simulink library "BESS_lib"  (Simulink 8.1)
settings: Solver=ode45  SolverMode=SingleTasking  StartTime=0.0  StopTime=10.0  RelTol=1e-3
undefined symbols (not defined in the file or in its folder): DiscIntNeverNeededParam, gcbh, sps_rtmsupport, Ts
libraries: simulink x25, powerlib x6, powerlib_meascontrol x4, powerlib_extras x3, simulink_extras x1, debounce_lib x1
(part 2 of 2)

== system BESS_lib/NREL_BESS/Protection/bitwise_faults ==
  note: Constant array has LSB on most left.
  S : Inport
  Bitwise Operator : simulink/Logic and Bit Operations/Bitwise Operator  logicop=OR  UseBitMask=off  NumInputPorts=8  BitMask=bin2dec('11011001')  BitMaskRealWorld=Stored Integer
  Data Type Conversion : DataTypeConversion  OutDataTypeStr=uint16
  Data Type Conversion1 : DataTypeConversion  OutDataTypeStr=double
  Demux : Demux  Outputs=8
  Shift Arithmetic : ArithShift  BitShiftNumber=1  BitShiftDirection=Left
  Shift Arithmetic1 : ArithShift  BitShiftNumber=2  BitShiftDirection=Left
  Shift Arithmetic2 : ArithShift  BitShiftNumber=3  BitShiftDirection=Left
  Shift Arithmetic3 : ArithShift  BitShiftNumber=4  BitShiftDirection=Left
  Shift Arithmetic4 : ArithShift  BitShiftNumber=5  BitShiftDirection=Left
  Shift Arithmetic5 : ArithShift  BitShiftNumber=6  BitShiftDirection=Left
  Shift Arithmetic6 : ArithShift  BitShiftNumber=7  BitShiftDirection=Left
  s : Outport
  wires:
  Shift Arithmetic6/1 -> Bitwise Operator/8
  Demux/8 -> Shift Arithmetic6/1
  Shift Arithmetic5/1 -> Bitwise Operator/7
  Shift Arithmetic4/1 -> Bitwise Operator/6
  Shift Arithmetic3/1 -> Bitwise Operator/5
  Shift Arithmetic2/1 -> Bitwise Operator/4
  Shift Arithmetic1/1 -> Bitwise Operator/3
  Shift Arithmetic/1 -> Bitwise Operator/2
  Demux/7 -> Shift Arithmetic5/1
  Demux/6 -> Shift Arithmetic4/1
  Demux/5 -> Shift Arithmetic3/1
  Demux/4 -> Shift Arithmetic2/1
  Demux/3 -> Shift Arithmetic1/1
  Demux/2 -> Shift Arithmetic/1
  Demux/1 -> Bitwise Operator/1
  Data Type Conversion1/1 -> s/1
  Bitwise Operator/1 -> Data Type Conversion1/1
  S/1 -> Data Type Conversion/1
  Data Type Conversion/1 -> Demux/1

== system BESS_lib/NREL_BESS/Protection/bitwise_status ==
  note: Constant array has LSB on most left.
  S : Inport
  Bitwise Operator : simulink/Logic and Bit Operations/Bitwise Operator  logicop=OR  UseBitMask=off  NumInputPorts=3  BitMask=bin2dec('11011001')  BitMaskRealWorld=Stored Integer
  Data Type Conversion : DataTypeConversion  OutDataTypeStr=uint16
  Data Type Conversion1 : DataTypeConversion  OutDataTypeStr=double
  Demux : Demux  Outputs=3
  Shift Arithmetic : ArithShift  BitShiftNumber=1  BitShiftDirection=Left
  Shift Arithmetic1 : ArithShift  BitShiftNumber=2  BitShiftDirection=Left
  s : Outport
  wires:
  Data Type Conversion/1 -> Demux/1
  S/1 -> Data Type Conversion/1
  Bitwise Operator/1 -> Data Type Conversion1/1
  Data Type Conversion1/1 -> s/1
  Demux/1 -> Bitwise Operator/1
  Demux/2 -> Shift Arithmetic/1
  Demux/3 -> Shift Arithmetic1/1
  Shift Arithmetic/1 -> Bitwise Operator/2
  Shift Arithmetic1/1 -> Bitwise Operator/3

== system BESS_lib/NREL_BESS/Ref_Limiting/RefLimiting ==
  fvpq_in : Inport
  p_max : Inport  Port=2
  p_min : Inport  Port=3
  Complex to Magnitude-Angle : ComplexToMagnitudeAngle
  Complex to Real-Imag : ComplexToRealImag
  Demux : Demux
  Magnitude-Angle to Complex : MagnitudeAngleToComplex
  Mux2 : Mux
  Real-Imag to Complex : RealImagToComplex
  Saturation : Saturate  UpperLimit=1.1  LowerLimit=0.9
  Saturation Dynamic : simulink/Discontinuities/Saturation Dynamic  OutMin=[]  OutMax=[]  OutDataTypeStr=Inherit: Same as second input  OutDataType=fixdt(1, 16)  OutScaling=2^-10  DoSatur=off
  Saturation1 : Saturate  UpperLimit=1.1  LowerLimit=0.9
  Saturation2 : Saturate  UpperLimit=1  LowerLimit=0
  fvpq_out : Outport
  wires:
  p_min/1 -> Saturation Dynamic/3
  Saturation1/1 -> Mux2/2
  Magnitude-Angle to Complex/1 -> Complex to Real-Imag/1
  Mux2/1 -> fvpq_out/1  "fvpq"
  Demux/3 -> Saturation Dynamic/2
  Saturation Dynamic/1 -> Real-Imag to Complex/1
  Complex to Magnitude-Angle/1 -> Saturation2/1
  Complex to Real-Imag/2 -> Mux2/4
  Complex to Real-Imag/1 -> Mux2/3
  Real-Imag to Complex/1 -> Complex to Magnitude-Angle/1
  Demux/2 -> Saturation1/1
  Demux/1 -> Saturation/1
  fvpq_in/1 -> Demux/1
  Saturation2/1 -> Magnitude-Angle to Complex/1
  Saturation/1 -> Mux2/1
  p_max/1 -> Saturation Dynamic/1
  Complex to Magnitude-Angle/2 -> Magnitude-Angle to Complex/2
  Demux/4 -> Real-Imag to Complex/2

== system BESS_lib/NREL_BESS/Inverter Controller/rate_limit/RateLimitwRst ==
  Rst : Inport
  In : Inport  Port=2
  Constant : Constant  Value=0
  Saturation : Saturate  UpperLimit=Ts*BP.I_slewrate  LowerLimit=-Ts*BP.I_slewrate
  Sum : Sum  Inputs=-+|
  Sum1 : Sum  Inputs=|++
  Switch : Switch  Criteria=u2 > Threshold  Threshold=0.5
  Unit Delay : UnitDelay  SampleTime=Ts
  Out : Outport
  wires:
  Sum1/1 -> Switch/3
  Saturation/1 -> Sum1/1
  Rst/1 -> Switch/2
  Switch/1 -> Unit Delay/1
  Constant/1 -> Switch/1
  Unit Delay/1 -> Out/1, Sum/1, Sum1/2
  Sum/1 -> Saturation/1
  In/1 -> Sum/2

== system BESS_lib/NREL_BESS/Inverter Controller/rate_limit/RateLimitwRst1 ==
  Rst : Inport
  In : Inport  Port=2
  Constant : Constant  Value=0
  Saturation : Saturate  UpperLimit=Ts*BP.I_slewrate  LowerLimit=-Ts*BP.I_slewrate
  Sum : Sum  Inputs=-+|
  Sum1 : Sum  Inputs=|++
  Switch : Switch  Criteria=u2 > Threshold  Threshold=0.5
  Unit Delay : UnitDelay  SampleTime=Ts
  Out : Outport
  wires:
  In/1 -> Sum/2
  Sum/1 -> Saturation/1
  Unit Delay/1 -> Sum1/2, Sum/1, Out/1
  Constant/1 -> Switch/1
  Switch/1 -> Unit Delay/1
  Rst/1 -> Switch/2
  Saturation/1 -> Sum1/1
  Sum1/1 -> Switch/3

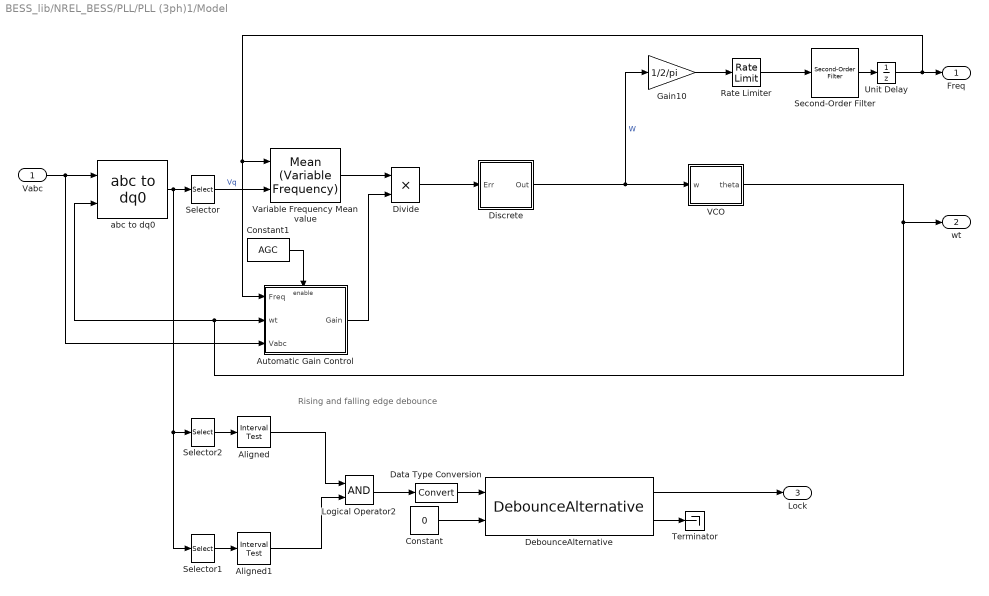
== system BESS_lib/NREL_BESS/PLL/PLL (3ph)1/Model ==
  note: Rising and falling edge debounce
  Vabc : Inport  PortDimensions=3
  Aligned : simulink/Logic and Bit Operations/Interval Test  IntervalClosedRight=on  uplimit=0.05  IntervalClosedLeft=on  lowlimit=-0.05  OutDataTypeStr=boolean
  Aligned1 : simulink/Logic and Bit Operations/Interval Test  IntervalClosedRight=on  uplimit=1.25  IntervalClosedLeft=on  lowlimit=0.05  OutDataTypeStr=boolean
  Automatic Gain Control : Subsystem  TreatAsAtomicUnit=on
  Constant : Constant  Value=0
  Constant1 : Constant  Value=AGC  SampleTime=Ts
  Data Type Conversion : DataTypeConversion
  DebounceAlternative : debounce_lib/DebounceAlternative  Tdb_off=0.5  Tdb_on=4  Tdb_sample=Tc
  Discrete : Subsystem  DialogController=POWERSYS.PowerSysDialog  VariantControl=PID_Discrete  mask(Discrete PID Controller){Kp=ParK(1), Ki=ParK(2), Kd=ParK(3), TcD=TcD, Par_Limits=[Flim(2) Flim(1)]*2*pi, Init=2*pi*Par_Init(2), Ts=Ts}
      mask prompts: Kp "Proportional gain (Kp):"; Ki "Integral gain (Ki):"; Kd "Derivative gain (Kd):"; TcD "Time constant for derivative filter (s):"; Par_Limits "Output limits: [ Upper   Lower ]"; Init "Output initial value:"; Ts "Sample time:"
      mask help: This block implements a discrete PID controller.
      mask Display: disp('PID');
  Divide : Product
  Gain10 : Gain  Gain=1/2/pi  SaturateOnIntegerOverflow=on  OutDataTypeStr=Inherit: Same as input  ParamDataTypeStr=Inherit: Same as input
  Logical Operator2 : Logic  AllPortsSameDT=off  OutDataTypeStr=boolean
  Rate Limiter : RateLimiter  RisingSlewLimit=MaxRateChangeFreq  FallingSlewLimit=-MaxRateChangeFreq  SampleTimeMode=inherited  InitialCondition=Par_Init(2)
  Second-Order Filter : powerlib_meascontrol/Filters/Second-Order Filter  FilterType=Lowpass  Fo=FilterCutOffFreq  Zeta=0.707  Ts=Ts  Initialize=on  Vac_Init=[0 0 Par_Init(2)]  Vdc_Init=Par_Init(2)  PlotResponse=off  FreqRange=[1 500 1]
  Selector : Selector  InputPortWidth=3  IndexOptions=Index vector (dialog)  Indices=2  OutputSizes=1
  Selector1 : Selector  InputPortWidth=3  IndexOptions=Index vector (dialog)  Indices=1  OutputSizes=1
  Selector2 : Selector  InputPortWidth=3  IndexOptions=Index vector (dialog)  Indices=2  OutputSizes=1
  Terminator : Terminator
  Unit Delay : UnitDelay  InitialCondition=Par_Init(2)  SampleTime=Ts
  VCO : Subsystem
  Variable Frequency Mean value : powerlib_meascontrol/Measurements/Mean (Variable Frequency)  Finit=Par_Init(2)  Fmin=Flim(1)  Vinit=0  Ts=Ts
  abc to dq0 : powerlib_meascontrol/Transformations/abc to dq0  Alignment=90 degrees behind phase A axis
  Freq : Outport
  wt : Outport  Port=2
  Lock : Outport  Port=3
  wires:
  VCO/1(theta) -> abc to dq0/2, Automatic Gain Control/2(wt), wt/1
  Data Type Conversion/1 -> DebounceAlternative/1
  Constant/1 -> DebounceAlternative/2
  DebounceAlternative/2 -> Terminator/1
  Logical Operator2/1 -> Data Type Conversion/1
  Selector2/1 -> Aligned/1
  Selector1/1 -> Aligned1/1
  Aligned1/1 -> Logical Operator2/2
  Aligned/1 -> Logical Operator2/1
  DebounceAlternative/1 -> Lock/1
  Discrete/1(Out) -> VCO/1(w), Gain10/1  "W"
  Unit Delay/1 -> Freq/1, Automatic Gain Control/1(Freq), Variable Frequency Mean value/1
  Rate Limiter/1 -> Second-Order Filter/1
  Gain10/1 -> Rate Limiter/1
  Selector/1 -> Variable Frequency Mean value/2  "Vq"
  Second-Order Filter/1 -> Unit Delay/1
  abc to dq0/1 -> Selector/1, Selector1/1, Selector2/1
  Vabc/1 -> abc to dq0/1, Automatic Gain Control/3(Vabc)
  Variable Frequency Mean value/1 -> Divide/1
  Automatic Gain Control/1(Gain) -> Divide/2
  Divide/1 -> Discrete/1(Err)
  Constant1/1 -> Automatic Gain Control/Enable

== system BESS_lib/NREL_BESS/Protection/Fault_Latch/SR_Prior_S ==
  S : Inport
  R : Inport  Port=2
  Logical Operator2 : Logic  Operator=OR  AllPortsSameDT=off  OutDataTypeStr=boolean
  Logical Operator3 : Logic  AllPortsSameDT=off  OutDataTypeStr=boolean
  Logical Operator4 : Logic  Operator=NOT  AllPortsSameDT=off  OutDataTypeStr=boolean
  Memory : Memory
  Q : Outport
  wires:
  Logical Operator3/1 -> Logical Operator2/2
  Memory/1 -> Logical Operator3/1, Q/1
  S/1 -> Logical Operator2/1
  Logical Operator4/1 -> Logical Operator3/2
  R/1 -> Logical Operator4/1
  Logical Operator2/1 -> Memory/1

== system BESS_lib/NREL_BESS/PLL/PLL (3ph)1/Model/Automatic Gain Control ==
  Freq : Inport
  wt : Inport  Port=2
  Vabc : Inport  Port=3
  Enable : EnablePort  PropagateVarSize=During execution
  Math Function : Math  Operator=reciprocal  SaturateOnIntegerOverflow=on
  Positive-Sequence (PLL-Driven) : powerlib_meascontrol/Measurements/Positive-Sequence (PLL-Driven)  Finit=Par_Init(2)  Fmin=Flim(1)  InInit=[1 0]  Ts=Ts
  Saturation : Saturate  UpperLimit=inf  LowerLimit=eps
  Terminator1 : Terminator
  Gain : Outport  InitialOutput=[1]
  wires:
  Positive-Sequence (PLL-Driven)/1 -> Saturation/1
  Positive-Sequence (PLL-Driven)/2 -> Terminator1/1
  wt/1 -> Positive-Sequence (PLL-Driven)/2
  Math Function/1 -> Gain/1
  Vabc/1 -> Positive-Sequence (PLL-Driven)/3
  Freq/1 -> Positive-Sequence (PLL-Driven)/1
  Saturation/1 -> Math Function/1

== system BESS_lib/NREL_BESS/PLL/PLL (3ph)1/Model/Discrete ==
  note: Use internal or external tuning parameters
  Err : Inport  SampleTime=Ts
  Bus Selector1 : BusSelector  OutputSignals=pll_kp
  Bus Selector2 : BusSelector  OutputSignals=pll_ki
  Constant : Constant  Value=ExtTuningEna
  Constant1 : Constant  Value=Kp
  Constant2 : Constant  Value=ExtTuningEna
  Constant3 : Constant  Value=Ki
  "Discrete Derivative " : DiscreteTransferFcn  Numerator="[ 1  -1 ]*Kd"  Denominator="[ TcD  Ts-TcD ]"  SampleTime=Ts
  Discrete-Time Integrator : DiscreteIntegrator  gainval=1  InitialCondition=Init  SampleTime=Ts  LimitOutput=on  UpperSaturationLimit=Par_Limits(1)  LowerSaturationLimit=Par_Limits(2)  ICPrevOutput=DiscIntNeverNeededParam  ICPrevScaledInput=DiscIntNeverNeededParam
  Index Vector : MultiPortSwitch  DataPortOrder=Zero-based contiguous  Inputs=2  zeroidx=on
  Index Vector1 : MultiPortSwitch  DataPortOrder=Zero-based contiguous  Inputs=2  zeroidx=on
  Product : Product
  Product1 : Product
  Saturation1 : Saturate  UpperLimit=Par_Limits(1)  LowerLimit=Par_Limits(2)  SampleTime=Ts
  Sum6 : Sum  Inputs=+++  SampleTime=Ts  SaturateOnIntegerOverflow=on  InputSameDT=on  OutDataTypeStr=Inherit: Same as first input
  Out : Outport  SampleTime=Ts  InitialOutput=0
  wires:
  Constant3/1 -> Index Vector1/2
  Bus Selector2/1 -> Index Vector1/3  "<pll_ki>"
  [tuning] -> Bus Selector2/1
  Constant2/1 -> Index Vector1/1
  Constant1/1 -> Index Vector/2
  Bus Selector1/1 -> Index Vector/3  "<pll_kp>"
  [tuning] -> Bus Selector1/1
  Constant/1 -> Index Vector/1
  Index Vector/1 -> Product/1  "Kp"
  Index Vector1/1 -> Product1/2  "Ki"
  Product1/1 -> Discrete-Time Integrator/1
  "Discrete Derivative "/1 -> Sum6/3
  Discrete-Time Integrator/1 -> Sum6/2
  Product/1 -> Sum6/1
  Sum6/1 -> Saturation1/1
  Err/1 -> "Discrete Derivative "/1, Product/2, Product1/1
  Saturation1/1 -> Out/1

== system BESS_lib/NREL_BESS/PLL/PLL (3ph)1/Model/VCO ==
  w : Inport
  Compare To Constant : simulink/Logic and Bit Operations/Compare To Constant  relop=>=  const=pi  OutDataTypeStr=uint8
  Gain : Gain  Gain=2*pi  OutDataTypeStr=double
  Gain2 : Gain  Gain=Ts  SaturateOnIntegerOverflow=on  OutDataTypeStr=Inherit: Same as input  ParamDataTypeStr=Inherit: Same as input
  Sum : Sum  Inputs=-++
  Unit Delay1 : UnitDelay  SampleTime=-1
  theta : Outport
  wires:
  Sum/1 -> Unit Delay1/1
  Gain2/1 -> Sum/2
  Unit Delay1/1 -> theta/1, Sum/3, Compare To Constant/1  "wt"
  Compare To Constant/1 -> Gain/1
  Gain/1 -> Sum/1
  w/1 -> Gain2/1
